simulink model "gm_INTERLOCK_DELAY"  (R2016a)
settings: Solver=FixedStepDiscrete  StartTime=0.0  StopTime=10.0  RelTol=1e-3
libraries: simulink x6
settings Model: Creator=zedboard  LastModifiedBy=Wendel
settings OptimizationCC: BlockReduction=off  ConditionallyExecuteInputs=off  DefaultParameterBehavior=Inlined
settings DebuggingCC: AlgebraicLoopMsg=error  InheritedTsInSrcMsg=none
settings HardwareCC: ProdBitPerPointer=32  ProdLargestAtomicFloat=None  ProdIntDivRoundTo=Undefined  ProdEndianess=Unspecified  ProdWordSize=32  ProdHWDeviceType=ASIC/FPGA->ASIC/FPGA  ProdEqTarget=off

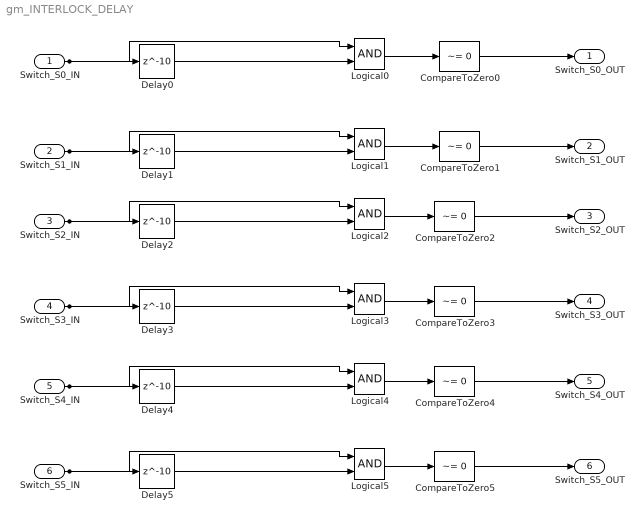
== system gm_INTERLOCK_DELAY ==
  Switch_S0_IN : Inport  OutDataTypeStr=boolean  SampleTime=0.001
  Switch_S1_IN : Inport  Port=2  OutDataTypeStr=boolean  SampleTime=0.001
  Switch_S2_IN : Inport  Port=3  OutDataTypeStr=boolean  SampleTime=0.001
  Switch_S3_IN : Inport  Port=4  OutDataTypeStr=boolean  SampleTime=0.001
  Switch_S4_IN : Inport  Port=5  OutDataTypeStr=boolean  SampleTime=0.001
  Switch_S5_IN : Inport  Port=6  OutDataTypeStr=boolean  SampleTime=0.001
  CompareToZero{0..5} (6 alike) : simulink/Logic and Bit Operations/Compare To Zero  relop=~=  OutDataTypeStr=boolean
  Delay0 : Delay  DelayLength=10  InitialCondition=0  SampleTime=0.001
  Delay{1..5} (5 alike) : Delay  DelayLength=10  InitialCondition=0
  Logical{0..5} (6 alike) : Logic  AllPortsSameDT=off  OutDataTypeStr=boolean
  Switch_S0_OUT : Outport
  Switch_S1_OUT : Outport  Port=2
  Switch_S2_OUT : Outport  Port=3
  Switch_S3_OUT : Outport  Port=4
  Switch_S4_OUT : Outport  Port=5
  Switch_S5_OUT : Outport  Port=6
  wires:
  Switch_S0_IN/1 -> Logical0/1, Delay0/1
  Switch_S1_IN/1 -> Logical1/1, Delay1/1
  Switch_S2_IN/1 -> Logical2/1, Delay2/1
  Switch_S3_IN/1 -> Logical3/1, Delay3/1
  Switch_S4_IN/1 -> Logical4/1, Delay4/1
  Switch_S5_IN/1 -> Logical5/1, Delay5/1
  CompareToZero0/1 -> Switch_S0_OUT/1
  CompareToZero1/1 -> Switch_S1_OUT/1
  CompareToZero2/1 -> Switch_S2_OUT/1
  CompareToZero3/1 -> Switch_S3_OUT/1
  CompareToZero4/1 -> Switch_S4_OUT/1
  CompareToZero5/1 -> Switch_S5_OUT/1
  Delay0/1 -> Logical0/2
  Delay1/1 -> Logical1/2
  Delay2/1 -> Logical2/2
  Delay3/1 -> Logical3/2
  Delay4/1 -> Logical4/2
  Delay5/1 -> Logical5/2
  Logical0/1 -> CompareToZero0/1
  Logical1/1 -> CompareToZero1/1
  Logical2/1 -> CompareToZero2/1
  Logical3/1 -> CompareToZero3/1
  Logical4/1 -> CompareToZero4/1
  Logical5/1 -> CompareToZero5/1
